simulink model "sim_PID"  (R2019b)
settings: Solver=VariableStepAuto  StartTime=0.0  StopTime=10  RelTol=1e-3
values from neighbouring files (symbols this model uses):
  LA = (uN*alfa_5*T_prima-rho*Cd*vN*A)/m    (= -0.0101244052863)    [coefficients.m]
  LB = alfa_5*Tm*(1-beta*(alfa_5*vN/wm -1)^2)/m    (= 1.32030612245)    [coefficients.m]
  t_c = -g*cos(theta_N)/(LB) *(slope_grades*pi/180)    [coefficients.m]
  Ts = 0.01    [coefficients.m]    (also in discretizar_C.m)
  uN = (m*g*Cr+rho*Cd*A*(vN^2)/2)/(alfa_5*T_alpha_n_v)    (= 0.168748744107)    [coefficients.m]
  vN = 20    [coefficients.m]
undefined symbols (not defined in the file or in its folder): k_CC, k_CD, k_GD, p_CC, p_CD, p_GD, z_CC, z_CD, z_GD
settings Model: Creator=Esteban  LastModifiedBy=Esteban

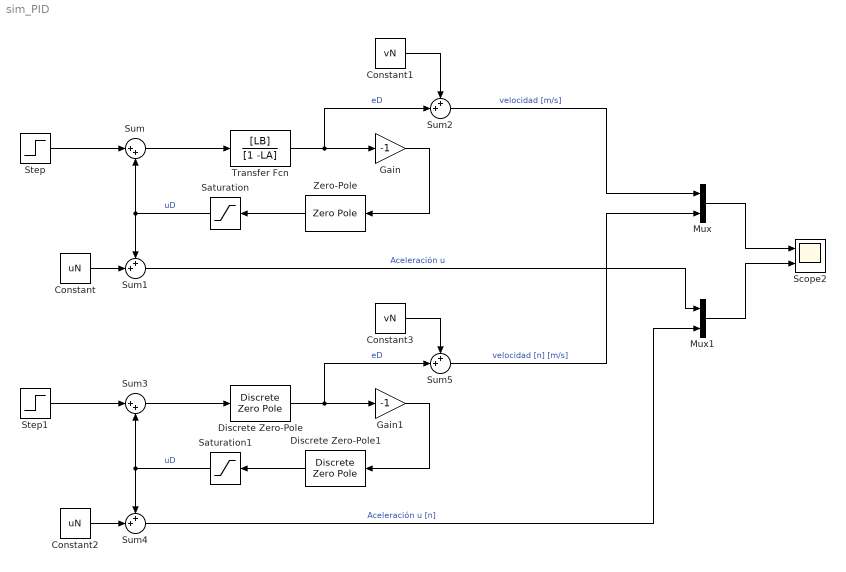
== system sim_PID ==
  Constant : Constant  Value=uN
  Constant1 : Constant  Value=vN
  Constant2 : Constant  Value=uN
  Constant3 : Constant  Value=vN
  Discrete Zero-Pole : DiscreteZeroPole  Zeros=[z_GD{:,1}]  Poles=[p_GD{:,1}]  Gain=k_GD  SampleTime=Ts
  Discrete Zero-Pole1 : DiscreteZeroPole  Zeros=[z_CD{:,1}]  Poles=[p_CD{:,1}]  Gain=k_CD  SampleTime=Ts
  Gain : Gain  Gain=-1
  Gain1 : Gain  Gain=-1
  Mux : Mux  Inputs=2
  Mux1 : Mux  Inputs=2
  Saturation : Saturate  UpperLimit=1-uN  LowerLimit=-uN
  Saturation1 : Saturate  UpperLimit=1-uN  LowerLimit=-uN
  Scope2 : Scope  NumInputPorts=2
  Step : Step  After=t_c  SampleTime=0
  Step1 : Step  After=t_c  SampleTime=Ts
  Sum : Sum  Inputs=|++
  Sum{1..2,4..5} (4 alike) : Sum  Inputs=++|
  Sum3 : Sum  Inputs=|++
  Transfer Fcn : TransferFcn  Numerator=[LB]  Denominator=[1 -LA]
  Zero-Pole : ZeroPole  Zeros=[z_CC{:,1}]  Poles=[p_CC{:,1}]  Gain=[k_CC]
  wires:
  Sum/1 -> Transfer Fcn/1
  Transfer Fcn/1 -> Sum2/2, Gain/1  "eD"
  Zero-Pole/1 -> Saturation/1
  Step/1 -> Sum/1
  Gain/1 -> Zero-Pole/1
  Constant/1 -> Sum1/2
  Sum1/1 -> Mux1/1  "Aceleración u"
  Constant1/1 -> Sum2/1
  Sum2/1 -> Mux/1  "velocidad [m/s]"
  Saturation/1 -> Sum1/1, Sum/2  "uD"
  Constant3/1 -> Sum5/1
  Sum4/1 -> Mux1/2  "Aceleración u [n]"
  Gain1/1 -> Discrete Zero-Pole1/1
  Constant2/1 -> Sum4/2
  Sum5/1 -> Mux/2  "velocidad [n] [m/s]"
  Sum3/1 -> Discrete Zero-Pole/1
  Step1/1 -> Sum3/1
  Discrete Zero-Pole/1 -> Sum5/2, Gain1/1  "eD"
  Saturation1/1 -> Sum4/1, Sum3/2  "uD"
  Discrete Zero-Pole1/1 -> Saturation1/1
  Mux/1 -> Scope2/1
  Mux1/1 -> Scope2/2
